simulink model "pH_Level_Detection_and_Regulation"  (R2022a)
settings: Solver=FixedStepAuto  StartTime=0.0  StopTime=inf  RelTol=1e-3
libraries: arduinolib x5, simulink x3
settings Model: ExtModeTrigDuration=2  Creator=AJ Dave  LastModifiedBy=Zero Two
settings SolverCC: AutoInsertRateTranBlk=on
settings OptimizationCC: EnhancedBackFolding=on  PassReuseOutputArgsAs=Individual arguments  ZeroExternalMemoryAtStartup=off  ZeroInternalMemoryAtStartup=off  MaxStackSize=64  OptimizeBlockOrder=speed  DifferentSizesBufferReuse=on  OptimizationCustomize=off  EfficientTunableParamExpr=on
settings DebuggingCC: ParameterTunabilityLossMsg=error
settings HardwareCC: ProdBitPerInt=16  ProdBitPerPointer=16  ProdBitPerSizeT=16  ProdBitPerPtrDiffT=16  ProdLargestAtomicFloat=None  ProdWordSize=8  ProdHWDeviceType=Atmel->AVR  UseEmbeddedCoderFeatures=off
settings ModelReferenceCC: EnableRefExpFcnMdlSchedulingChecks=off
settings SFSimCC: MATLABDynamicMemAlloc=off
settings RTWCC: SystemTargetFile=ert.tlc  HardwareBoard=Arduino Uno  TemplateMakefile=ert_default_tmf  Toolchain=Arduino AVR  GPUComputeCapability=5.0
settings CodeAppCC: ForceParamTrailComments=on  IgnoreCustomStorageClasses=off  OperatorAnnotations=on  SimulinkDataObjDesc=on  SFDataObjDesc=on  InsertBlockDesc=on
settings ERTTargetCC: SupportContinuousTime=on  SupportNonInlinedSFcns=on  SupportVariableSizeSignals=on  ExtModeTransport=3  ExtModeStaticAlloc=on  ExtModeStaticAllocSize=250  ExtModeMexFile=ext_xcp  ExtModeIntrfLevel=Level2 - Open

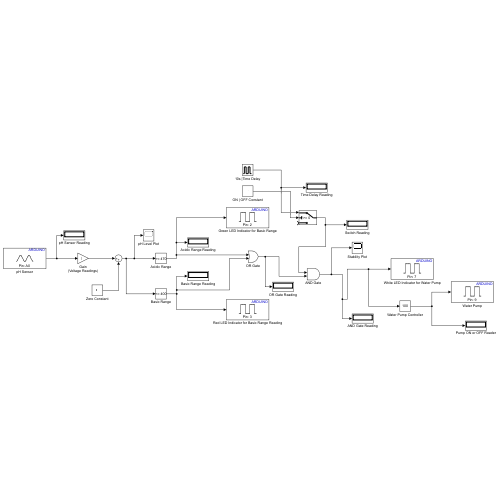
[thumbnail: Simulink's stored preview of the top-level diagram]
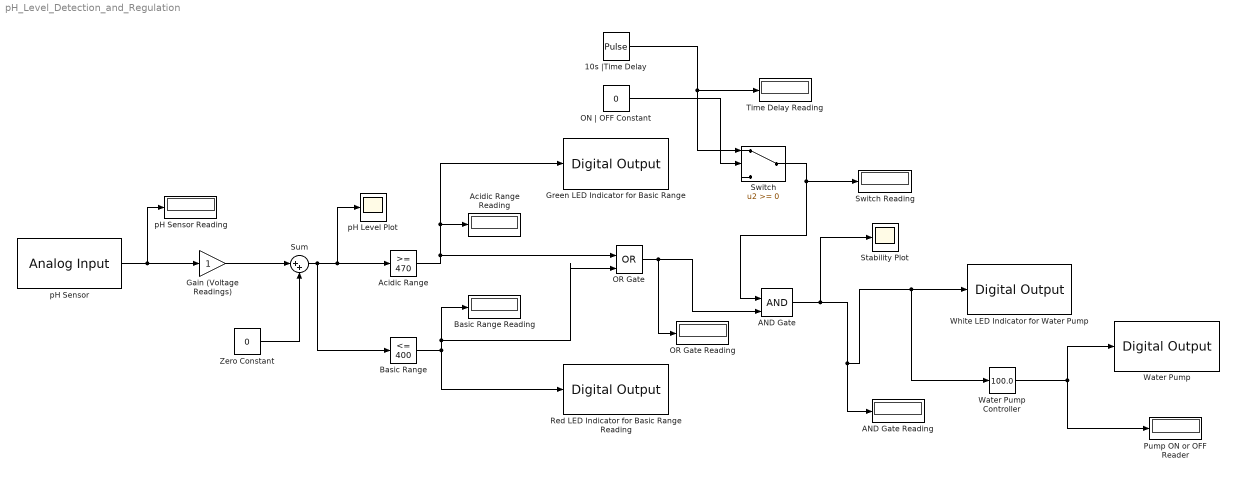
== system pH_Level_Detection_and_Regulation ==
  10s |Time Delay : DiscretePulseGenerator  PulseType=Time based  Period=10  PulseWidth=50
  AND Gate : Logic  IconShape=distinctive  AllPortsSameDT=off  OutDataTypeStr=boolean
  AND Gate Reading : Display
  Acidic Range : simulink/Logic and Bit Operations/Compare To Constant  relop=>=  const=470  OutDataTypeStr=boolean
  Acidic Range Reading : Display
  Basic Range : simulink/Logic and Bit Operations/Compare To Constant  relop=<=  const=400  OutDataTypeStr=boolean
  Basic Range Reading : Display
  Gain (Voltage Readings) : Gain
  Green LED Indicator for Basic Range : arduinolib/Digital Output  pinNumber=2  Direction=output  blockPlatform=arduino
  ON | OFF Constant : Constant  Value=0
  OR Gate : Logic  Operator=OR  IconShape=distinctive  AllPortsSameDT=off  OutDataTypeStr=boolean
  OR Gate Reading : Display
  Pump ON or OFF Reader : Display
  Red LED Indicator for Basic Range Reading : arduinolib/Digital Output  pinNumber=3  Direction=output  blockPlatform=arduino
  Stability Plot : Scope
  Sum : Sum  Inputs=|++
  Switch : Switch  SaturateOnIntegerOverflow=off  InputSameDT=off
  Switch Reading : Display
  Time Delay Reading : Display
  Water Pump : arduinolib/Digital Output  pinNumber=9  Direction=output  blockPlatform=arduino
  Water Pump Controller : simulink/Math Operations/Slider Gain  gain=100.0  low=0  high=100
  White LED Indicator for Water Pump : arduinolib/Digital Output  pinNumber=7  Direction=output  blockPlatform=arduino
  Zero Constant : Constant  Value=0
  pH Level Plot : Scope
  pH Sensor : arduinolib/Analog Input  pinNumber=0  ReadResultsOnly=off  ConversionTriggerSource=Software  ExternalTriggerType=uint32( 0 )  OutputDataType=uint16  EnableConversionCompleteNotify=off  EnableOuputStatus=off  SampleTime=0.03  blockPlatform=arduino
  pH Sensor Reading : Display
  wires:
  pH Sensor/1 -> pH Sensor Reading/1, Gain (Voltage Readings)/1
  Gain (Voltage Readings)/1 -> Sum/1
  Sum/1 -> Basic Range/1, pH Level Plot/1, Acidic Range/1
  Zero Constant/1 -> Sum/2
  Acidic Range/1 -> Green LED Indicator for Basic Range/1, Acidic Range Reading/1, OR Gate/1
  Basic Range/1 -> Basic Range Reading/1, OR Gate/2, Red LED Indicator for Basic Range Reading/1
  OR Gate/1 -> OR Gate Reading/1, AND Gate/2
  Water Pump Controller/1 -> Pump ON or OFF Reader/1, Water Pump/1
  10s |Time Delay/1 -> Switch/1, Time Delay Reading/1
  ON | OFF Constant/1 -> Switch/2
  Switch/1 -> AND Gate/1, Switch Reading/1
  AND Gate/1 -> Stability Plot/1, AND Gate Reading/1, Water Pump Controller/1, White LED Indicator for Water Pump/1
